simulink model "Copy_of_PID_Validation"  (R2024b)
settings: Solver=ode45  StartTime=0.0  StopTime=10  RelTol=1e-3
InitFcn:
  | Init
values from neighbouring files (symbols this model uses):
  Beq_p = 1.41e-6    (= 1.41e-06)    [Init.m]
  k_drv = (1 + drv.R3/drv.R4) * drv.R2/(drv.R1 + drv.R2)    [Init.m]
  Kd = Kp * Td    [Init.m]
  Ki = Kp / Ti    [Init.m]
  Kp = deltak * cos(deltaphi)    [Init.m]
  Kw = 1/Tw    (= 33.3333333333)    [Init.m]
  rpm2degs = 360/60    (= 6)    [Init.m]
  rpm2rads = 2*pi/60    (= 0.10471975512)    [Init.m]
  tau_sf_p = 7.02e-3    (= 0.00702)    [Init.m]
  tl = 1/(3*wgc)    [Init.m]
undefined symbols (not defined in the file or in its folder): drv, gbox, mld, mot, sens
libraries: simulink_extras x1, simulink x1
settings Model: Creator=Banaan  LastModifiedBy=lucag

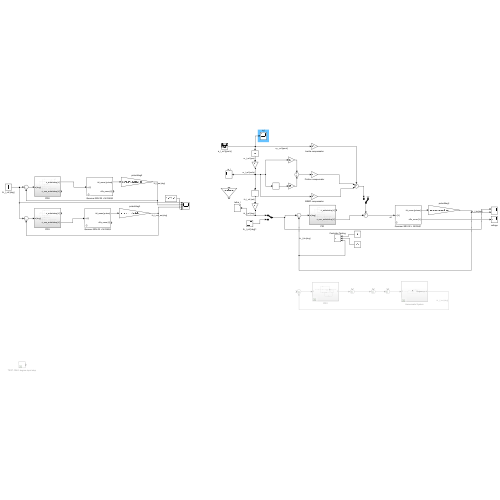
[thumbnail: Simulink's stored preview of the top-level diagram]
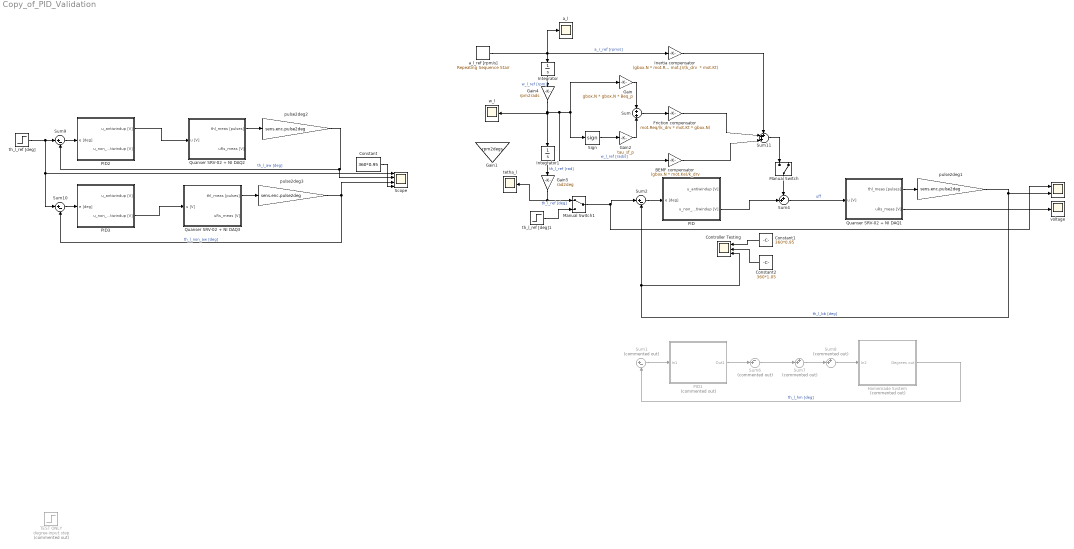
== system Copy_of_PID_Validation ==
  " " : Scope  NumInputPorts=2
  " a_l" : Scope
  " tetha_l" : Scope
  " w_l" : Scope
  BEMF compensator : Gain  Gain=(gbox.N * mot.Ke)/k_drv
  Constant : Constant  Value=360*0.95
  Constant1 : Constant  Value=360*0.95
  Constant2 : Constant  Value=360*1.05
  Controller Testing : Scope  NumInputPorts=3
  Friction compensator : Gain  Gain=mot.Req/(k_drv * mot.Kt * gbox.N)
  Gain : Gain  Gain=gbox.N * gbox.N * Beq_p
  Gain1 : Gain  Gain=rpm2degs
  Gain2 : Gain  Gain=tau_sf_p
  Gain4 : Gain  Gain=rpm2rads
  Gain5 : Gain  Gain=rad2deg
  Homemade System : Subsystem  Commented=on
  Inertia compensator : Gain  Gain="(gbox.N * mot.Req * mot.J)/(k_drv  * mot.Kt)"
  Integrator : Integrator
  Integrator1 : Integrator
  Manual Switch : ManualSwitch  CurrentSetting=0
  Manual Switch1 : ManualSwitch
  PID : Subsystem
  PID1 : Subsystem  Commented=on
  PID2 : Subsystem
  PID3 : Subsystem
  Quanser SRV-02 + NI DAQ1 : Subsystem  mask(Quanser SRV-02 (with inertial load) + NI DAQ){Ts=0.001, fricType=Coulomb + viscous}
      mask prompts: Ts "NI DAQ Sample Time:"; fricType "Friction model"
      mask help: Quanser SRV-02 (with inertial load) + NI DAQ model.
      mask init:
      | %%  Sensors data
      | 
      | %   shunt resistor
      | sens.curr.Rs = 0.5;                         %   resistance [Ohm]   
      | sens.curr.uRs_std = 0.01;                   %   voltage noise standard dev [V]                           
      | sens.curr.uRs_var = sens.curr.uRs_std^2;	%   voltage noise variance [V^2]
      | 
      | %   Hewlett-Packard HEDS-5540#A06 optical encoder
      | sens.enc.ppr = 500*4;                       %   pulses per rotation
      | sens.enc.pulse2deg = 360/sens.enc.ppr;      %   [pulses] -> [deg]
      | sens.enc.pulse2rad = 2*pi/sens.enc.ppr;     %   [pulses] -> [rad]
      | sens.enc.deg2pulse = sens.enc.ppr/360;      %   [deg] -> [pulses]
      | sens.enc.rad2pulse = sens.enc.ppr/2/pi;     %   [rad] -> [pulses]
      | 
      | 
      | %%  Data acquisition board (daq) data
      | 
      | %   NI PCI-6221 DAC data
      | daq.dac.bits = 16;                                  %   resolution (bits)
      | daq.dac.fs   = 10;                                  %   full scale 
      | daq.dac.q    = 2*daq.dac.fs/(2^daq.dac.bits-1);     %	quantization
      | 
      | %   NI PCI-6221 ADC data
      | daq.adc.bits = 16;                                  %   resolution (bits)
      | daq.adc.fs   = 10;                                  %   full scale (as set in SLDRT Analog Input block)
      | daq.adc.q    = 2*daq.adc.fs/(2^daq.adc.bits-1);     %   quantization
      mask Help:
      | Riccardo Antonello (antonello@dei.unipd.it)
      | 
      | April 24, 2020
      | 
      | Dept. of Information Engineering, University of Padova
      mask TypeOptions fricType: Coulomb + viscous | Karnopp
  Quanser SRV-02 + NI DAQ2 : Subsystem  mask(Quanser SRV-02 (with inertial load) + NI DAQ){Ts=0.001, fricType=Coulomb + viscous}
      mask prompts: Ts "NI DAQ Sample Time:"; fricType "Friction model"
      mask help: Quanser SRV-02 (with inertial load) + NI DAQ model.
      mask init: same as Copy_of_PID_Validation/Quanser SRV-02 + NI DAQ1
      mask Help:
      | Riccardo Antonello (antonello@dei.unipd.it)
      | 
      | April 24, 2020
      | 
      | Dept. of Information Engineering, University of Padova
      mask TypeOptions fricType: Coulomb + viscous | Karnopp
  Quanser SRV-02 + NI DAQ3 : Subsystem  mask(Quanser SRV-02 (with inertial load) + NI DAQ){Ts=0.001, fricType=Coulomb + viscous}
      mask prompts: Ts "NI DAQ Sample Time:"; fricType "Friction model"
      mask help: Quanser SRV-02 (with inertial load) + NI DAQ model.
      mask init: same as Copy_of_PID_Validation/Quanser SRV-02 + NI DAQ1
      mask Help:
      | Riccardo Antonello (antonello@dei.unipd.it)
      | 
      | April 24, 2020
      | 
      | Dept. of Information Engineering, University of Padova
      mask TypeOptions fricType: Coulomb + viscous | Karnopp
  Scope : Scope  NumInputPorts=4
  Sign : Signum
  Sum : Sum  Inputs=+|+
  Sum1 : Sum  Commented=on  Inputs=|+-
  Sum10 : Sum  Inputs=|+-
  Sum11 : Sum  Inputs=+++|
  Sum2 : Sum  Inputs=|+-
  Sum4 : Sum  Inputs=++|
  Sum6 : Sum  Commented=on  Inputs=-+|
  Sum7 : Sum  Commented=on  Inputs=++|
  Sum8 : Sum  Commented=on  Inputs=++|
  Sum9 : Sum  Inputs=|+-
  TEST ONLY degree-input step : Step  Commented=on  After=360  SampleTime=0
  a_l_ref [rpm/s] : simulink/Sources/Repeating Sequence Stair  OutValues=[900 0 -900 -900 0 900]  tsamp=0.5  OutMin=[]  OutMax=[]  OutDataTypeStr=double  OutputDataTypeScalingMode=double  OutDataType=fixdt(0,8)  ConRadixGroup=Best Precision: Vector-wise  OutScaling=2^-12
  pulse2deg1 : Gain  Gain=sens.enc.pulse2deg
  pulse2deg2 : Gain  Gain=sens.enc.pulse2deg
  pulse2deg3 : Gain  Gain=sens.enc.pulse2deg
  th_l_ref [deg] : Step  After=360  SampleTime=0
  th_l_ref [deg]1 : Step  After=360  SampleTime=0
  voltage : Scope
  wires:
  Constant1/1 -> Controller Testing/1
  Sum2/1 -> PID/1(e [deg])
  Quanser SRV-02 + NI DAQ1/1(thl_meas [pulses]) -> pulse2deg1/1
  Constant2/1 -> Controller Testing/2
  Quanser SRV-02 + NI DAQ1/2(uRs_meas [V]) -> voltage/1
  pulse2deg1/1 -> Sum2/2, Controller Testing/3, " "/2  "th_l_bb [deg]"
  Sum1/1 -> PID1/1(In1)
  Homemade System/1(Degrees out) -> Sum1/2  "th_l_hm [deg]"
  Integrator1/1 -> Gain5/1  "th_l_ref [rad]"
  Gain/1 -> Sum/1
  Sum/1 -> Friction compensator/1
  Sum4/1 -> Quanser SRV-02 + NI DAQ1/1(u [V])  "uff"
  PID1/1(Out1) -> Sum6/2
  Sum6/1 -> Sum7/2
  Sum7/1 -> Sum8/2
  Sum8/1 -> Homemade System/1(In2)
  Sign/1 -> Gain2/1
  Gain2/1 -> Sum/2
  Integrator/1 -> Gain4/1  "w_l_ref [rpm]"
  Sum9/1 -> PID2/1(e [deg])
  PID2/1(u_antiwindup [V]) -> Quanser SRV-02 + NI DAQ2/1(u [V])
  Quanser SRV-02 + NI DAQ2/1(thl_meas [pulses]) -> pulse2deg2/1
  Quanser SRV-02 + NI DAQ3/1(thl_meas [pulses]) -> pulse2deg3/1
  Sum10/1 -> PID3/1(e [deg])
  pulse2deg2/1 -> Scope/2, Sum9/2  "th_l_aw [deg]"
  PID3/2(u_non_antiwindup [V]) -> Quanser SRV-02 + NI DAQ3/1(u [V])
  pulse2deg3/1 -> Scope/3, Sum10/2  "th_l_non_aw [deg]"
  th_l_ref [deg]/1 -> Sum10/1, Scope/1, Sum9/1
  Gain4/1 -> BEMF compensator/1, Sign/1, Gain/1, Integrator1/1, " w_l"/1  "w_l_ref [rad/s]"
  Gain5/1 -> Manual Switch1/1, " tetha_l"/1  "th_l_ref [deg]"
  a_l_ref [rpm/s]/1 -> " a_l"/1, Inertia compensator/1, Integrator/1  "a_r_ref [rpm/s]"
  BEMF compensator/1 -> Sum11/3
  Friction compensator/1 -> Sum11/2
  Inertia compensator/1 -> Sum11/1
  Sum11/1 -> Manual Switch/1
  Manual Switch/1 -> Sum4/1
  Manual Switch1/1 -> " "/1, Sum2/1
  th_l_ref [deg]1/1 -> Manual Switch1/2
  Constant/1 -> Scope/4
  PID/2(u_non_antiwindup [V]) -> Sum4/2

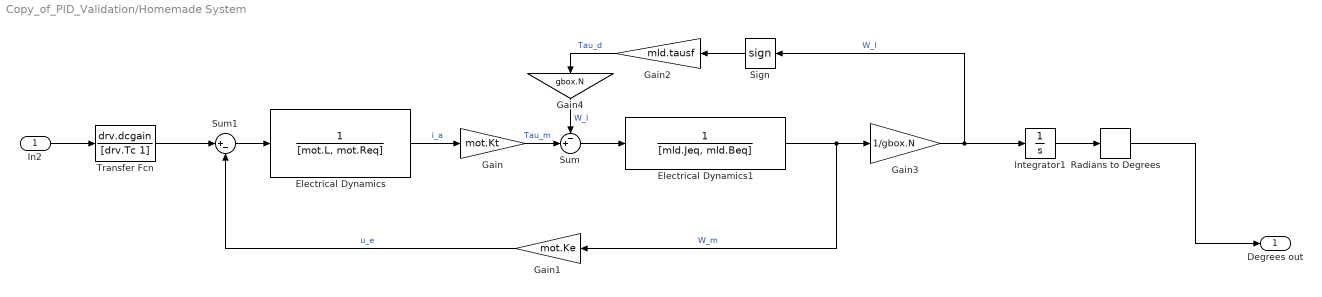
== system Copy_of_PID_Validation/Homemade System ==
  In2 : Inport
  Electrical Dynamics : TransferFcn  Denominator=[mot.L, mot.Req]
  Electrical Dynamics1 : TransferFcn  Denominator=[mld.Jeq, mld.Beq]
  Gain : Gain  Gain=mot.Kt
  Gain1 : Gain  Gain=mot.Ke
  Gain2 : Gain  Gain=mld.tausf
  Gain3 : Gain  Gain=1/gbox.N
  Gain4 : Gain  Gain=gbox.N
  Integrator1 : Integrator
  Radians to Degrees : simulink_extras/Transformations/Radians to Degrees
  Sign : Signum  ZeroCross=off
  Sum : Sum  Inputs=-+|
  Sum1 : Sum  Inputs=|+-
  Transfer Fcn : TransferFcn  Numerator=drv.dcgain  Denominator=[drv.Tc 1]
  Degrees out : Outport
  wires:
  Gain/1 -> Sum/2  "Tau_m"
  Electrical Dynamics1/1 -> Gain1/1, Gain3/1  "W_m"
  Integrator1/1 -> Radians to Degrees/1
  Gain3/1 -> Integrator1/1, Sign/1  "W_l"
  Sign/1 -> Gain2/1
  Gain1/1 -> Sum1/2  "u_e"
  Electrical Dynamics/1 -> Gain/1  "i_a"
  Gain4/1 -> Sum/1  "W_l"
  Sum/1 -> Electrical Dynamics1/1
  Gain2/1 -> Gain4/1  "Tau_d"
  Sum1/1 -> Electrical Dynamics/1
  Transfer Fcn/1 -> Sum1/1
  Radians to Degrees/1 -> Degrees out/1
  In2/1 -> Transfer Fcn/1

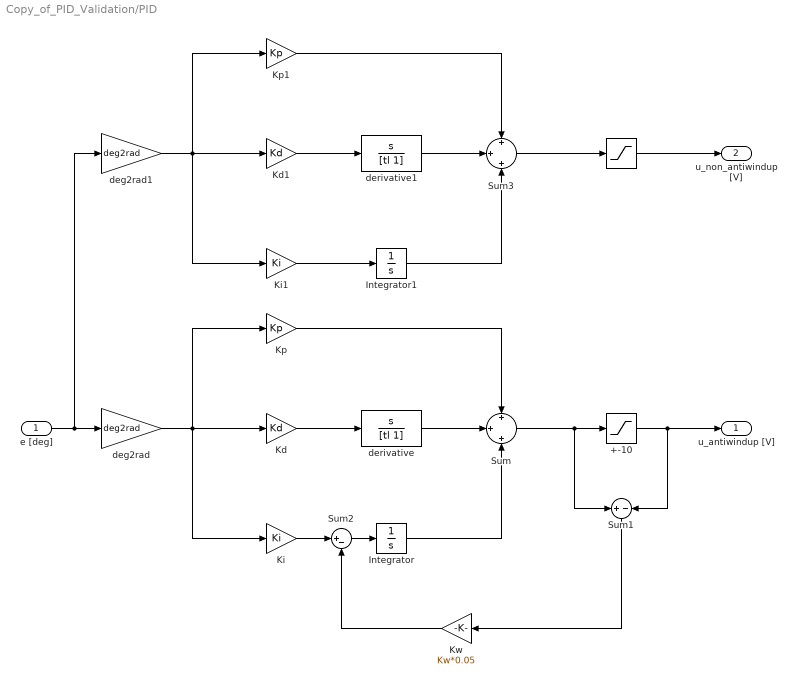
== system Copy_of_PID_Validation/PID ==
  e [deg] : Inport
  " " : Saturate  UpperLimit=10  LowerLimit=-10
  +-10 : Saturate  UpperLimit=10  LowerLimit=-10
  Integrator : Integrator
  Integrator1 : Integrator
  Kd : Gain  Gain=Kd
  Kd1 : Gain  Gain=Kd
  Ki : Gain  Gain=Ki
  Ki1 : Gain  Gain=Ki
  Kp : Gain  Gain=Kp
  Kp1 : Gain  Gain=Kp
  Kw : Gain  Gain=Kw*0.05
  Sum : Sum  Inputs=+|+|+
  Sum1 : Sum  Inputs=+|-
  Sum2 : Sum  Inputs=|+-
  Sum3 : Sum  Inputs=+|+|+
  deg2rad : Gain  Gain=deg2rad
  deg2rad1 : Gain  Gain=deg2rad
  derivative : TransferFcn  Numerator=[1 0]  Denominator=[tl 1]
  derivative1 : TransferFcn  Numerator=[1 0]  Denominator=[tl 1]
  u_antiwindup [V] : Outport
  u_non_antiwindup [V] : Outport  Port=2
  wires:
  e [deg]/1 -> deg2rad1/1, deg2rad/1
  deg2rad/1 -> Kp/1, Ki/1, Kd/1
  Ki/1 -> Sum2/1
  Kp/1 -> Sum/1
  Integrator/1 -> Sum/3
  Kd/1 -> derivative/1
  derivative/1 -> Sum/2
  Sum/1 -> Sum1/1, +-10/1
  Sum2/1 -> Integrator/1
  Sum1/1 -> Kw/1
  Kw/1 -> Sum2/2
  +-10/1 -> u_antiwindup [V]/1, Sum1/2
  deg2rad1/1 -> Kp1/1, Ki1/1, Kd1/1
  Sum3/1 -> " "/1
  derivative1/1 -> Sum3/2
  Kd1/1 -> derivative1/1
  Ki1/1 -> Integrator1/1
  Kp1/1 -> Sum3/1
  Integrator1/1 -> Sum3/3
  " "/1 -> u_non_antiwindup [V]/1

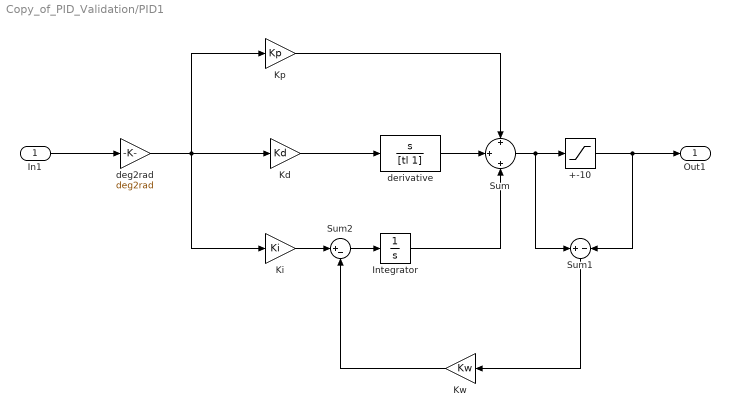
== system Copy_of_PID_Validation/PID1 ==
  In1 : Inport
  +-10 : Saturate  UpperLimit=10  LowerLimit=-10
  Integrator : Integrator
  Kd : Gain  Gain=Kd
  Ki : Gain  Gain=Ki
  Kp : Gain  Gain=Kp
  Kw : Gain  Gain=Kw
  Sum : Sum  Inputs=+|+|+
  Sum1 : Sum  Inputs=+|-
  Sum2 : Sum  Inputs=|+-
  deg2rad : Gain  Gain=deg2rad
  derivative : TransferFcn  Numerator=[1 0]  Denominator=[tl 1]
  Out1 : Outport
  wires:
  Kd/1 -> derivative/1
  Kp/1 -> Sum/1
  Ki/1 -> Sum2/1
  deg2rad/1 -> Kp/1, Kd/1, Ki/1
  In1/1 -> deg2rad/1
  Sum1/1 -> Kw/1
  +-10/1 -> Sum1/2, Out1/1
  Sum/1 -> Sum1/1, +-10/1
  Integrator/1 -> Sum/3
  derivative/1 -> Sum/2
  Sum2/1 -> Integrator/1
  Kw/1 -> Sum2/2

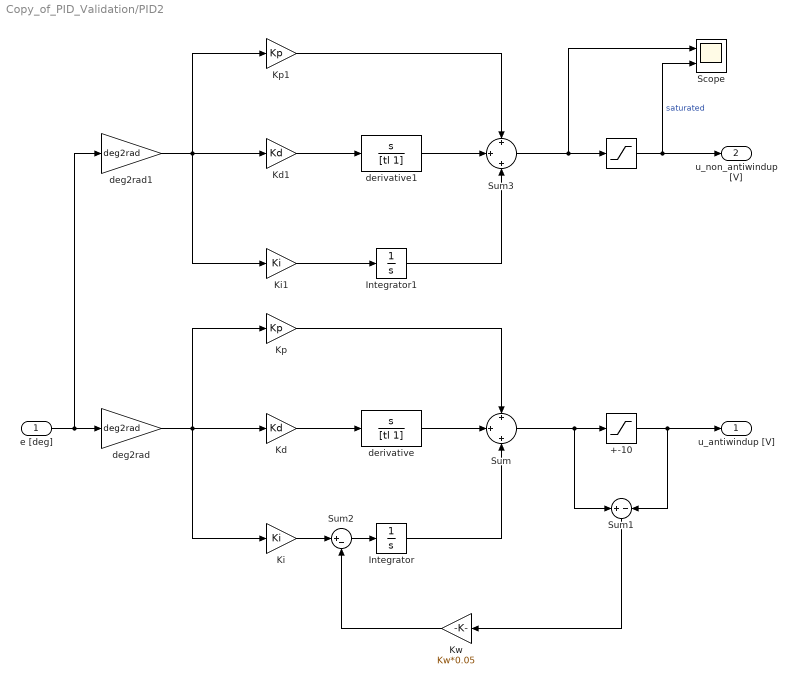
== system Copy_of_PID_Validation/PID2 ==
  e [deg] : Inport
  " " : Saturate  UpperLimit=10  LowerLimit=-10
  +-10 : Saturate  UpperLimit=10  LowerLimit=-10
  Integrator : Integrator
  Integrator1 : Integrator
  Kd : Gain  Gain=Kd
  Kd1 : Gain  Gain=Kd
  Ki : Gain  Gain=Ki
  Ki1 : Gain  Gain=Ki
  Kp : Gain  Gain=Kp
  Kp1 : Gain  Gain=Kp
  Kw : Gain  Gain=Kw*0.05
  Scope : Scope  NumInputPorts=2
  Sum : Sum  Inputs=+|+|+
  Sum1 : Sum  Inputs=+|-
  Sum2 : Sum  Inputs=|+-
  Sum3 : Sum  Inputs=+|+|+
  deg2rad : Gain  Gain=deg2rad
  deg2rad1 : Gain  Gain=deg2rad
  derivative : TransferFcn  Numerator=[1 0]  Denominator=[tl 1]
  derivative1 : TransferFcn  Numerator=[1 0]  Denominator=[tl 1]
  u_antiwindup [V] : Outport
  u_non_antiwindup [V] : Outport  Port=2
  wires:
  " "/1 -> Scope/2, u_non_antiwindup [V]/1  "saturated"
  Integrator1/1 -> Sum3/3
  Kp1/1 -> Sum3/1
  Ki1/1 -> Integrator1/1
  Kd1/1 -> derivative1/1
  derivative1/1 -> Sum3/2
  Sum3/1 -> Scope/1, " "/1
  deg2rad1/1 -> Kd1/1, Ki1/1, Kp1/1
  +-10/1 -> Sum1/2, u_antiwindup [V]/1
  Kw/1 -> Sum2/2
  Sum1/1 -> Kw/1
  Sum2/1 -> Integrator/1
  Sum/1 -> +-10/1, Sum1/1
  derivative/1 -> Sum/2
  Kd/1 -> derivative/1
  Integrator/1 -> Sum/3
  Kp/1 -> Sum/1
  Ki/1 -> Sum2/1
  deg2rad/1 -> Kd/1, Ki/1, Kp/1
  e [deg]/1 -> deg2rad/1, deg2rad1/1

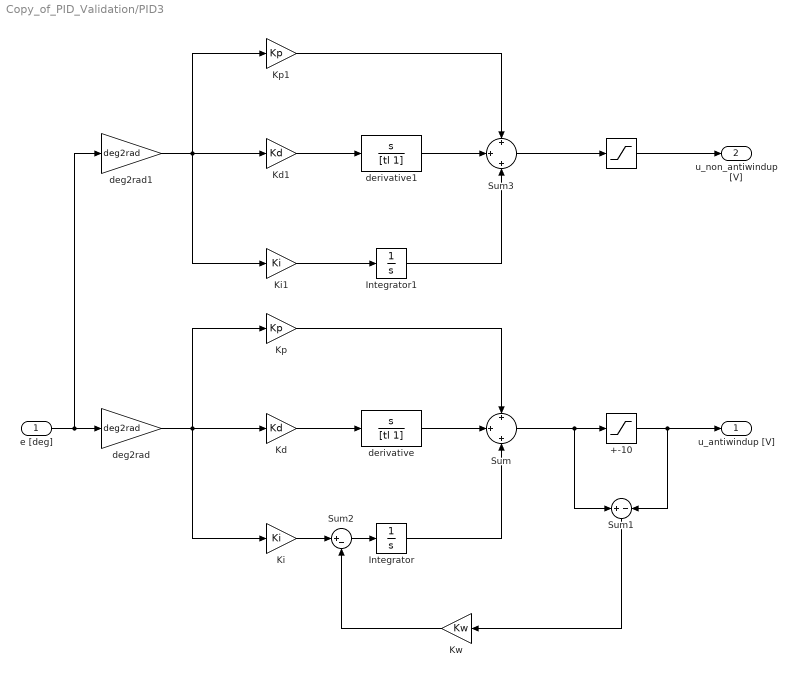
== system Copy_of_PID_Validation/PID3 ==
  e [deg] : Inport
  " " : Saturate  UpperLimit=10  LowerLimit=-10
  +-10 : Saturate  UpperLimit=10  LowerLimit=-10
  Integrator : Integrator
  Integrator1 : Integrator
  Kd : Gain  Gain=Kd
  Kd1 : Gain  Gain=Kd
  Ki : Gain  Gain=Ki
  Ki1 : Gain  Gain=Ki
  Kp : Gain  Gain=Kp
  Kp1 : Gain  Gain=Kp
  Kw : Gain  Gain=Kw
  Sum : Sum  Inputs=+|+|+
  Sum1 : Sum  Inputs=+|-
  Sum2 : Sum  Inputs=|+-
  Sum3 : Sum  Inputs=+|+|+
  deg2rad : Gain  Gain=deg2rad
  deg2rad1 : Gain  Gain=deg2rad
  derivative : TransferFcn  Numerator=[1 0]  Denominator=[tl 1]
  derivative1 : TransferFcn  Numerator=[1 0]  Denominator=[tl 1]
  u_antiwindup [V] : Outport
  u_non_antiwindup [V] : Outport  Port=2
  wires:
  e [deg]/1 -> deg2rad1/1, deg2rad/1
  deg2rad/1 -> Kp/1, Ki/1, Kd/1
  Ki/1 -> Sum2/1
  Kp/1 -> Sum/1
  Integrator/1 -> Sum/3
  Kd/1 -> derivative/1
  derivative/1 -> Sum/2
  Sum/1 -> Sum1/1, +-10/1
  Sum2/1 -> Integrator/1
  Sum1/1 -> Kw/1
  Kw/1 -> Sum2/2
  +-10/1 -> u_antiwindup [V]/1, Sum1/2
  deg2rad1/1 -> Kp1/1, Ki1/1, Kd1/1
  Sum3/1 -> " "/1
  derivative1/1 -> Sum3/2
  Kd1/1 -> derivative1/1
  Ki1/1 -> Integrator1/1
  Kp1/1 -> Sum3/1
  Integrator1/1 -> Sum3/3
  " "/1 -> u_non_antiwindup [V]/1

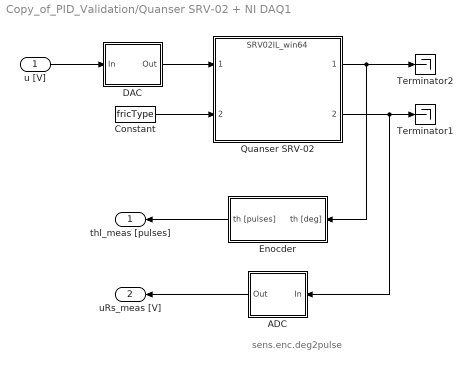
== system Copy_of_PID_Validation/Quanser SRV-02 + NI DAQ1 ==
  note: sens.enc.deg2pulse
  u [V] : Inport
  ADC : Subsystem
  Constant : Constant  Value=fricType
  DAC : Subsystem
  Enocder : Subsystem
  Quanser SRV-02 : ModelReference  ModelNameDialog=SRV02IL_win64.slxp  ModelReferenceVersion=1.44  CopyOfModelProtected=on
  Terminator1 : Terminator
  Terminator2 : Terminator
  thl_meas [pulses] : Outport
  uRs_meas [V] : Outport  Port=2
  wires:
  Enocder/1(th [pulses]) -> thl_meas [pulses]/1
  ADC/1(Out) -> uRs_meas [V]/1
  DAC/1(Out) -> Quanser SRV-02/1
  Quanser SRV-02/2 -> ADC/1(In), Terminator1/1
  u [V]/1 -> DAC/1(In)
  Quanser SRV-02/1 -> Enocder/1(th [deg]), Terminator2/1
  Constant/1 -> Quanser SRV-02/2

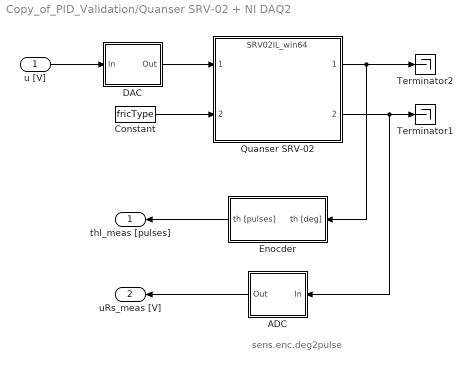
== system Copy_of_PID_Validation/Quanser SRV-02 + NI DAQ2 ==
  note: sens.enc.deg2pulse
  u [V] : Inport
  ADC : Subsystem
  Constant : Constant  Value=fricType
  DAC : Subsystem
  Enocder : Subsystem
  Quanser SRV-02 : ModelReference  ModelNameDialog=SRV02IL_win64.slxp  ModelReferenceVersion=1.44  CopyOfModelProtected=on
  Terminator1 : Terminator
  Terminator2 : Terminator
  thl_meas [pulses] : Outport
  uRs_meas [V] : Outport  Port=2
  wires:
  Constant/1 -> Quanser SRV-02/2
  Quanser SRV-02/1 -> Terminator2/1, Enocder/1(th [deg])
  u [V]/1 -> DAC/1(In)
  Quanser SRV-02/2 -> Terminator1/1, ADC/1(In)
  DAC/1(Out) -> Quanser SRV-02/1
  ADC/1(Out) -> uRs_meas [V]/1
  Enocder/1(th [pulses]) -> thl_meas [pulses]/1

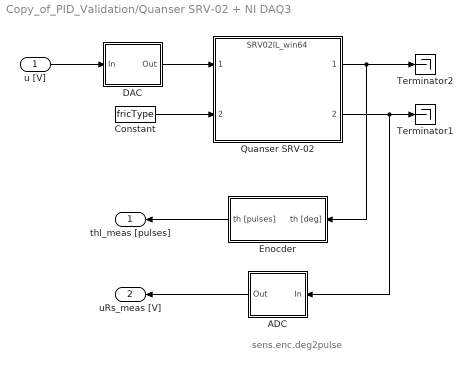
== system Copy_of_PID_Validation/Quanser SRV-02 + NI DAQ3 ==
  note: sens.enc.deg2pulse
  u [V] : Inport
  ADC : Subsystem
  Constant : Constant  Value=fricType
  DAC : Subsystem
  Enocder : Subsystem
  Quanser SRV-02 : ModelReference  ModelNameDialog=SRV02IL_win64.slxp  ModelReferenceVersion=1.44  CopyOfModelProtected=on
  Terminator1 : Terminator
  Terminator2 : Terminator
  thl_meas [pulses] : Outport
  uRs_meas [V] : Outport  Port=2
  wires:
  Enocder/1(th [pulses]) -> thl_meas [pulses]/1
  ADC/1(Out) -> uRs_meas [V]/1
  DAC/1(Out) -> Quanser SRV-02/1
  Quanser SRV-02/2 -> ADC/1(In), Terminator1/1
  u [V]/1 -> DAC/1(In)
  Quanser SRV-02/1 -> Enocder/1(th [deg]), Terminator2/1
  Constant/1 -> Quanser SRV-02/2

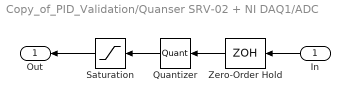
== system Copy_of_PID_Validation/Quanser SRV-02 + NI DAQ1/ADC ==
  In : Inport
  Quantizer : Quantizer  QuantizationInterval=daq.adc.q
  Saturation : Saturate  UpperLimit=daq.adc.fs  LowerLimit=-daq.adc.fs
  Zero-Order Hold : ZeroOrderHold  SampleTime=Ts
  Out : Outport
  wires:
  Saturation/1 -> Out/1
  In/1 -> Zero-Order Hold/1
  Quantizer/1 -> Saturation/1
  Zero-Order Hold/1 -> Quantizer/1

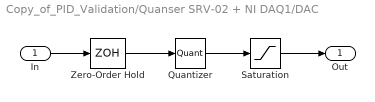
== system Copy_of_PID_Validation/Quanser SRV-02 + NI DAQ1/DAC ==
  In : Inport
  Quantizer : Quantizer  QuantizationInterval=daq.dac.q
  Saturation : Saturate  UpperLimit=daq.dac.fs  LowerLimit=-daq.dac.fs
  Zero-Order Hold : ZeroOrderHold  SampleTime=Ts
  Out : Outport
  wires:
  Quantizer/1 -> Saturation/1
  In/1 -> Zero-Order Hold/1
  Zero-Order Hold/1 -> Quantizer/1
  Saturation/1 -> Out/1

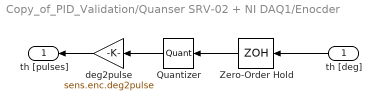
== system Copy_of_PID_Validation/Quanser SRV-02 + NI DAQ1/Enocder ==
  th [deg] : Inport
  Quantizer : Quantizer  QuantizationInterval=sens.enc.pulse2deg
  Zero-Order Hold : ZeroOrderHold  SampleTime=Ts
  deg2pulse : Gain  Gain=sens.enc.deg2pulse
  th [pulses] : Outport
  wires:
  Quantizer/1 -> deg2pulse/1
  th [deg]/1 -> Zero-Order Hold/1
  Zero-Order Hold/1 -> Quantizer/1
  deg2pulse/1 -> th [pulses]/1

== system Copy_of_PID_Validation/Quanser SRV-02 + NI DAQ2/ADC ==
  In : Inport
  Quantizer : Quantizer  QuantizationInterval=daq.adc.q
  Saturation : Saturate  UpperLimit=daq.adc.fs  LowerLimit=-daq.adc.fs
  Zero-Order Hold : ZeroOrderHold  SampleTime=Ts
  Out : Outport
  wires:
  Zero-Order Hold/1 -> Quantizer/1
  Quantizer/1 -> Saturation/1
  In/1 -> Zero-Order Hold/1
  Saturation/1 -> Out/1

== system Copy_of_PID_Validation/Quanser SRV-02 + NI DAQ2/DAC ==
  In : Inport
  Quantizer : Quantizer  QuantizationInterval=daq.dac.q
  Saturation : Saturate  UpperLimit=daq.dac.fs  LowerLimit=-daq.dac.fs
  Zero-Order Hold : ZeroOrderHold  SampleTime=Ts
  Out : Outport
  wires:
  Saturation/1 -> Out/1
  Zero-Order Hold/1 -> Quantizer/1
  In/1 -> Zero-Order Hold/1
  Quantizer/1 -> Saturation/1

== system Copy_of_PID_Validation/Quanser SRV-02 + NI DAQ2/Enocder ==
  th [deg] : Inport
  Quantizer : Quantizer  QuantizationInterval=sens.enc.pulse2deg
  Zero-Order Hold : ZeroOrderHold  SampleTime=Ts
  deg2pulse : Gain  Gain=sens.enc.deg2pulse
  th [pulses] : Outport
  wires:
  deg2pulse/1 -> th [pulses]/1
  Zero-Order Hold/1 -> Quantizer/1
  th [deg]/1 -> Zero-Order Hold/1
  Quantizer/1 -> deg2pulse/1

== system Copy_of_PID_Validation/Quanser SRV-02 + NI DAQ3/ADC ==
  In : Inport
  Quantizer : Quantizer  QuantizationInterval=daq.adc.q
  Saturation : Saturate  UpperLimit=daq.adc.fs  LowerLimit=-daq.adc.fs
  Zero-Order Hold : ZeroOrderHold  SampleTime=Ts
  Out : Outport
  wires:
  Saturation/1 -> Out/1
  In/1 -> Zero-Order Hold/1
  Quantizer/1 -> Saturation/1
  Zero-Order Hold/1 -> Quantizer/1

== system Copy_of_PID_Validation/Quanser SRV-02 + NI DAQ3/DAC ==
  In : Inport
  Quantizer : Quantizer  QuantizationInterval=daq.dac.q
  Saturation : Saturate  UpperLimit=daq.dac.fs  LowerLimit=-daq.dac.fs
  Zero-Order Hold : ZeroOrderHold  SampleTime=Ts
  Out : Outport
  wires:
  Quantizer/1 -> Saturation/1
  In/1 -> Zero-Order Hold/1
  Zero-Order Hold/1 -> Quantizer/1
  Saturation/1 -> Out/1

== system Copy_of_PID_Validation/Quanser SRV-02 + NI DAQ3/Enocder ==
  th [deg] : Inport
  Quantizer : Quantizer  QuantizationInterval=sens.enc.pulse2deg
  Zero-Order Hold : ZeroOrderHold  SampleTime=Ts
  deg2pulse : Gain  Gain=sens.enc.deg2pulse
  th [pulses] : Outport
  wires:
  Quantizer/1 -> deg2pulse/1
  th [deg]/1 -> Zero-Order Hold/1
  Zero-Order Hold/1 -> Quantizer/1
  deg2pulse/1 -> th [pulses]/1
